simulink model "four_bots_CNN_DSM_7"  (R2018b)
settings: Solver=ode5  StartTime=0.0  StopTime=20.0  FixedStep=0.0002  RelTol=1e-3
(part 2 of 2)

== matlab function four_bots_CNN_DSM_7/Multi agent System NN & SMC/Agent 3/MATLAB Function ==
  data: agent_x1 input; x2_dot output; agent_x2 input; t input; control_input input; fx_dt output
function [x2_dot, fx_dt] = physical_model( agent_x1 , agent_x2, t, control_input )

Mass=[4,5,4,5];
Alpha=[0.087,0.090,0.085,0.092];
Radius=[0.18,0.20,0.24,0.22];
Inertia=[0.12,0.15,0.13,0.14];
Beta=[11.4,11.6,11.8,12.0];

%% assign the parameter according to serial number
serial_num = 3; 

m=Mass(serial_num);
alpha=Alpha(serial_num);
R=Radius(serial_num);
inertia=Inertia(serial_num);
beta=Beta(serial_num);

%% current states of the robot
dimension=3;

theta=agent_x1(dimension);

%% the real model of robot
M=diag([1/m,1/m,1/inertia]);
T=[-sin(theta), -sin(pi/3-theta), sin(pi/3+theta);
    cos(theta), -cos(pi/3-theta), -cos(pi/3+theta);
    R,          R,                  R];

real_fx = -beta*M*(T*T')*agent_x2;
uncertain = [0.3*sin(0.5*t)+2; 0.2*cos(0.5*t)+1.5; 0.1*sin(0.3*t)+1];

%% saturation is added here for convinience
Vmax=6; % the maximum voltage of the motor

u1up=Vmax/(alpha*m)*(abs(sin(theta))+abs(sin(pi/3-theta))+abs(sin(pi/3+theta)));
u1do=-Vmax/(alpha*m)*(abs(sin(theta))+abs(sin(pi/3-theta))+abs(sin(pi/3+theta)));
u2up=Vmax/(alpha*m)*(abs(cos(theta))+abs(cos(pi/3-theta))+abs(cos(pi/3+theta)));
u2do=-Vmax/(alpha*m)*(abs(cos(theta))+abs(cos(pi/3-theta))+abs(cos(pi/3+theta)));
u3up=R/(alpha*inertia)*3*Vmax;
u3do=-R/(alpha*inertia)*3*Vmax;

control_input(1) = max( min(control_input(1),u1up), u1do );
control_input(2) = max( min(control_input(2),u2up), u2do );
control_input(3) = max( min(control_input(3),u3up), u3do );


fx_dt=real_fx + uncertain; 

x2_dot = real_fx + control_input + uncertain;


end

== matlab function four_bots_CNN_DSM_7/Multi agent System NN & SMC/Agent 3/MATLAB Function1 ==
  data: fx_dt input; esti_error output; fx_dtdot input; E input
function esti_error = estimation_error(fx_dt, fx_dtdot, E)

c=2.5;
lambda=2.5;

esti_error = fx_dtdot + (c + lambda) * fx_dt - E; 

end

== matlab function four_bots_CNN_DSM_7/Multi agent System NN & SMC/Agent 4/Controller /Chebyshev Polynomials ==
  data: current_states input; phi_x output
function phi_x = Chebyshev_polynomials(current_states)

%% parameters that may alter
dimension=3;
cheby_order=3;

%% current states
x1=current_states(dimension*0+1:dimension*1);
x2=current_states(dimension*1+1:dimension*2);

%% initialization
phi_x=ones(1+2*dimension*cheby_order,1);

%% recursion procedure
now_x=[x1;x2];
for order = 1 : cheby_order
   if order == 1
      phi_x(2*dimension*(order-1)+2:2*dimension*order+1)=now_x;
   elseif order == 2
      phi_x(2*dimension*(order-1)+2:2*dimension*order+1)=2*now_x.*phi_x(2*dimension*(order-2)+2:2*dimension*(order-1)+1)-1;
   else
      phi_x(2*dimension*(order-1)+2:2*dimension*order+1)=2*now_x.*phi_x(2*dimension*(order-2)+2:2*dimension*(order-1)+1)-phi_x(2*dimension*(order-3)+2:2*dimension*(order-2)+1);
   end
end

end

== matlab function four_bots_CNN_DSM_7/Multi agent System NN & SMC/Agent 4/Controller /Control dot ==
  data: L input; E input; xi input; error input; u_dot output; reference input; u input
function u_dot = control_dot(L, E, xi, error, reference, u)

%% parameters that may change
dimension=3;
c=2.5;
lambda=2.5;
eta=80;

serial_num=4;

num_agent=size(L,1); 
%% codes
r_acc=reference(dimension*num_agent*2+1 : dimension*num_agent*3);
r_accdot=reference(dimension*num_agent*3+1 : dimension*num_agent*4);

xd2_dot = r_acc(dimension*(serial_num-1)+1 : dimension*serial_num);
xd2_ddot = r_accdot(dimension*(serial_num-1)+1 : dimension*serial_num);

e2=error(dimension*1+1:dimension*2);

u_dot= -E + xd2_ddot + (c+lambda)*xd2_dot - (c+lambda)*u -c*lambda*e2 - eta*xi;

end

== matlab function four_bots_CNN_DSM_7/Multi agent System NN & SMC/Agent 4/Controller /Error Calculation ==
  data: cur_states output; current_states input; L input; error output; reference input
function [cur_states , error] = error_calculation(current_states, L, reference)

%% parameters that may change for alternative use
dimension=3;
serial_num=4;

num_agent=size(L,1);
%% current states
% get current states
pos=current_states(dimension*num_agent*0+1 : dimension*num_agent*1);
vol=current_states(dimension*num_agent*1+1 : dimension*num_agent*2);
acc=current_states(dimension*num_agent*2+1 : dimension*num_agent*3);

% get current reference
r_pos=reference(dimension*num_agent*0+1 : dimension*num_agent*1);
r_vol=reference(dimension*num_agent*1+1 : dimension*num_agent*2);
r_acc=reference(dimension*num_agent*2+1 : dimension*num_agent*3);

% agent j's states
agent_x1 = pos(dimension*(serial_num-1)+1 : dimension*serial_num);
agent_x2 = vol(dimension*(serial_num-1)+1 : dimension*serial_num);

% agent_x2dot = acc(dimension*(serial_num-1)+1 : dimension*serial_num);
% 
% % agent j's reference
% r_x1=r_pos(dimension*(serial_num-1)+1 : dimension*serial_num);
% r_x2=r_vol(dimension*(serial_num-1)+1 : dimension*serial_num);
% r_x2dot=r_acc(dimension*(serial_num-1)+1 : dimension*serial_num);

e_1 = kron(L(serial_num, : ), eye(dimension) ) * (pos - r_pos);
e_2 = kron(L(serial_num, : ), eye(dimension) ) * (vol - r_vol);
e_2dot = kron(L(serial_num, : ), eye(dimension) ) * (acc - r_acc);

cur_states = [agent_x1;agent_x2];
error = [e_1 ; e_2 ; e_2dot];

end

== matlab function four_bots_CNN_DSM_7/Multi agent System NN & SMC/Agent 4/Controller /Estimation ==
  data: phi_x input; W input; E output
function E = estimation(phi_x, W)
%% estimation
E=W'*phi_x;

end

== matlab function four_bots_CNN_DSM_7/Multi agent System NN & SMC/Agent 4/Controller /Parameter Tuning ==
  data: phi_x input; xi input; W_dot output
function W_dot = parameter_tuning(phi_x, xi)

%% parameters that may alter
dimension=3;
cheby_order=3;
F=0.1*eye(1+2*dimension*cheby_order);

%% codes
W_dot = F*phi_x*xi';

end

== matlab function four_bots_CNN_DSM_7/Multi agent System NN & SMC/Agent 4/Controller /Sliding Variable Generation ==
  data: error input; xi output
function xi = sliding_variable(error)

%% parameters that may alter
dimension=3;
c=2.5;
lambda=2.5;

%% codes
error_1=error(dimension*0+1:dimension*1);
error_2=error(dimension*1+1:dimension*2);
error_2dot=error(dimension*2+1:dimension*3);

xi = error_2dot + (c + lambda)* error_2 + lambda * c * error_1;

end

== matlab function four_bots_CNN_DSM_7/Multi agent System NN & SMC/Agent 4/Controller /neural_initial ==
  data: weight output
function weight = neural_initialize()

% cheby_order   : order of chebyshev polynomials
% dimension     : dimension of the system

cheby_order=3;
dimension=3;

weight = zeros(1+2*cheby_order*dimension, dimension);

end

== matlab function four_bots_CNN_DSM_7/Multi agent System NN & SMC/Agent 4/MATLAB Function ==
  data: agent_x1 input; x2_dot output; agent_x2 input; t input; control_input input; fx_dt output
function [x2_dot, fx_dt] = physical_model( agent_x1 , agent_x2, t, control_input )

Mass=[4,5,4,5];
Alpha=[0.087,0.090,0.085,0.092];
Radius=[0.18,0.20,0.24,0.22];
Inertia=[0.12,0.15,0.13,0.14];
Beta=[11.4,11.6,11.8,12.0];

%% assign the parameter according to serial number
serial_num = 4; 

m=Mass(serial_num);
alpha=Alpha(serial_num);
R=Radius(serial_num);
inertia=Inertia(serial_num);
beta=Beta(serial_num);

%% current states of the robot
dimension=3;

theta=agent_x1(dimension);

%% the real model of robot
M=diag([1/m,1/m,1/inertia]);
T=[-sin(theta), -sin(pi/3-theta), sin(pi/3+theta);
    cos(theta), -cos(pi/3-theta), -cos(pi/3+theta);
    R,          R,                  R];

real_fx = -beta*M*(T*T')*agent_x2;
uncertain = [0.3*sin(0.5*t)+2; 0.2*cos(0.5*t)+1.5; 0.1*sin(0.3*t)+1];

%% saturation is added here for convinience
Vmax=6; % the maximum voltage of the motor

u1up=Vmax/(alpha*m)*(abs(sin(theta))+abs(sin(pi/3-theta))+abs(sin(pi/3+theta)));
u1do=-Vmax/(alpha*m)*(abs(sin(theta))+abs(sin(pi/3-theta))+abs(sin(pi/3+theta)));
u2up=Vmax/(alpha*m)*(abs(cos(theta))+abs(cos(pi/3-theta))+abs(cos(pi/3+theta)));
u2do=-Vmax/(alpha*m)*(abs(cos(theta))+abs(cos(pi/3-theta))+abs(cos(pi/3+theta)));
u3up=R/(alpha*inertia)*3*Vmax;
u3do=-R/(alpha*inertia)*3*Vmax;

control_input(1) = max( min(control_input(1),u1up), u1do );
control_input(2) = max( min(control_input(2),u2up), u2do );
control_input(3) = max( min(control_input(3),u3up), u3do );


fx_dt=real_fx + uncertain; 

x2_dot = real_fx + control_input + uncertain;


end

== matlab function four_bots_CNN_DSM_7/Multi agent System NN & SMC/Agent 4/MATLAB Function1 ==
  data: fx_dt input; esti_error output; fx_dtdot input; E input
function esti_error = estimation_error(fx_dt, fx_dtdot, E)

c=2.5;
lambda=2.5;

esti_error = fx_dtdot + (c + lambda) * fx_dt - E; 

end

== matlab function four_bots_CNN_DSM_7/Reference Generator1/Acceleration reference ==
  data: t input; x2d_dot output
function x2d_dot = gene_ref_x2_dot(t)

%% generate position reference
radius=3;
w=0.1;
phase=-pi/4;

x1=[-radius*w^2*cos(w*t+pi/2*0+phase); -radius*w^2*sin(w*t+pi/2*0+phase); 0];
x2=[-radius*w^2*cos(w*t+pi/2*1+phase); -radius*w^2*sin(w*t+pi/2*1+phase); 0];
x3=[-radius*w^2*cos(w*t+pi/2*2+phase); -radius*w^2*sin(w*t+pi/2*2+phase); 0];
x4=[-radius*w^2*cos(w*t+pi/2*3+phase); -radius*w^2*sin(w*t+pi/2*3+phase); 0];

x2d_dot=[x1;x2;x3;x4];

== matlab function four_bots_CNN_DSM_7/Reference Generator1/Acceleration_dot Reference ==
  data: t input; x2ddot output
function x2ddot = gene_ref_x2ddot(t)

%% generate position reference
radius=3;
w=0.1;
phase=-pi/4;

x1=[radius*w^3*sin(w*t+pi/2*0+phase); -radius*w^3*cos(w*t+pi/2*0+phase); 0];
x2=[radius*w^3*sin(w*t+pi/2*1+phase); -radius*w^3*cos(w*t+pi/2*1+phase); 0];
x3=[radius*w^3*sin(w*t+pi/2*2+phase); -radius*w^3*cos(w*t+pi/2*2+phase); 0];
x4=[radius*w^3*sin(w*t+pi/2*3+phase); -radius*w^3*cos(w*t+pi/2*3+phase); 0];

x2ddot=[x1;x2;x3;x4];

== matlab function four_bots_CNN_DSM_7/Reference Generator1/Position Reference ==
  data: t input; x1d output
function x1d = gene_ref_x1(t)

%% generate position reference
radius=3;
w=0.1;
bias_x=0;
bias_y=0;
phase=-pi/4;

x1=[radius*cos(w*t+pi/2*0+phase)+bias_x ; radius*sin(w*t+pi/2*0+phase)+bias_y ; 0];
x2=[radius*cos(w*t+pi/2*1+phase)+bias_x ; radius*sin(w*t+pi/2*1+phase)+bias_y ; 0];
x3=[radius*cos(w*t+pi/2*2+phase)+bias_x ; radius*sin(w*t+pi/2*2+phase)+bias_y ; 0];
x4=[radius*cos(w*t+pi/2*3+phase)+bias_x ; radius*sin(w*t+pi/2*3+phase)+bias_y ; 0];

x1d=[x1;x2;x3;x4];

== matlab function four_bots_CNN_DSM_7/Reference Generator1/Speed Reference ==
  data: t input; x2d output
function x2d = gene_ref_x2(t)

%% generate position reference
radius=3;
w=0.1;
phase=-pi/4;

x1=[-radius*w*sin(w*t+pi/2*0+phase); radius*w*cos(w*t+pi/2*0+phase); 0];
x2=[-radius*w*sin(w*t+pi/2*1+phase); radius*w*cos(w*t+pi/2*1+phase); 0];
x3=[-radius*w*sin(w*t+pi/2*2+phase); radius*w*cos(w*t+pi/2*2+phase); 0];
x4=[-radius*w*sin(w*t+pi/2*3+phase); radius*w*cos(w*t+pi/2*3+phase); 0];

x2d=[x1;x2;x3;x4];

== matlab function four_bots_CNN_DSM_7/Multi agent System NN & SMC/Agent 3/Controller /Hysteresis/MATLAB Function1 ==
  data: u input; output output; u_dot input; zeta input; zeta_dot output
function [output,zeta_dot] = B_W_hysteresis(u, u_dot, zeta)

mu_1=1.5;
mu_2=3;
beta=1;
chi=0.5;
n=2;

output=mu_1*u+mu_2*zeta;

f=ones(3,1)-beta*sign(u_dot).*abs(zeta).^(n-1).*zeta-chi*abs(zeta).^n;

zeta_dot=u_dot.*f;
end

== matlab function four_bots_CNN_DSM_7/Multi agent System NN & SMC/Agent 3/Controller /Hysteresis/MATLAB Function2 ==
  data: u input; output output; u_dot input; zeta_1 input; zeta1_dot output
function [output,zeta1_dot] = inv_B_W_hysteresis(u, u_dot, zeta_1)

mu_1=1.5;
mu_2=3;
beta=1;
chi=0.5;
n=2;

output=1/mu_1*u - mu_2/mu_1*zeta_1;

f=ones(3,1)-beta*sign(u_dot/mu_1).*abs(zeta_1).^(n-1).*zeta_1-chi*abs(zeta_1).^n;

zeta1_dot=u_dot.*f./(mu_1+mu_2*f);
end

== matlab function four_bots_CNN_DSM_7/Multi agent System NN & SMC/Agent 1 /Controller /MATLAB Function ==
  data: W input; W output
function W = smooth_projection(W)

%% smooth projection
Wmax=0.3;
Wmin=-0.3;
epsi=0.01;

for i=1:size(W,1)
   for j=1:size(W,2)
      if W(i,j)>Wmax
          W(i,j)=Wmax + epsi * (1-exp(-(W(i,j)-Wmax)/epsi));
      elseif W(i,j)<Wmin
          W(i,j)=Wmin - epsi * (1-exp((W(i,j)-Wmin)/epsi));
      else
          W(i,j)=W(i,j);
      end
   end
end

end

== matlab function four_bots_CNN_DSM_7/Multi agent System NN & SMC/Agent 2/Controller /MATLAB Function ==
  data: W input; W output
function W = smooth_projection(W)

%% smooth projection
Wmax=0.3;
Wmin=-0.3;
epsi=0.01;

for i=1:size(W,1)
   for j=1:size(W,2)
      if W(i,j)>Wmax
          W(i,j)=Wmax + epsi * (1-exp(-(W(i,j)-Wmax)/epsi));
      elseif W(i,j)<Wmin
          W(i,j)=Wmin - epsi * (1-exp((W(i,j)-Wmin)/epsi));
      else
          W(i,j)=W(i,j);
      end
   end
end

end

== matlab function four_bots_CNN_DSM_7/Multi agent System NN & SMC/Agent 4/Controller /Hysteresis1/MATLAB Function1 ==
  data: u input; output output; u_dot input; zeta input; zeta_dot output
function [output,zeta_dot] = B_W_hysteresis(u, u_dot, zeta)

mu_1=1.5;
mu_2=3;
beta=1;
chi=0.5;
n=2;

output=mu_1*u+mu_2*zeta;

f=ones(3,1)-beta*sign(u_dot).*abs(zeta).^(n-1).*zeta-chi*abs(zeta).^n;

zeta_dot=u_dot.*f;
end

== matlab function four_bots_CNN_DSM_7/Multi agent System NN & SMC/Agent 4/Controller /Hysteresis1/MATLAB Function2 ==
  data: u input; output output; u_dot input; zeta_1 input; zeta1_dot output
function [output,zeta1_dot] = inv_B_W_hysteresis(u, u_dot, zeta_1)

mu_1=1.5;
mu_2=3;
beta=1;
chi=0.5;
n=2;

output=1/mu_1*u - mu_2/mu_1*zeta_1;

f=ones(3,1)-beta*sign(u_dot/mu_1).*abs(zeta_1).^(n-1).*zeta_1-chi*abs(zeta_1).^n;

zeta1_dot=u_dot.*f./(mu_1+mu_2*f);
end

== matlab function four_bots_CNN_DSM_7/Multi agent System NN & SMC/Agent 3/Controller /MATLAB Function ==
  data: W input; W output
function W = smooth_projection(W)

%% smooth projection
Wmax=0.3;
Wmin=-0.3;
epsi=0.01;

for i=1:size(W,1)
   for j=1:size(W,2)
      if W(i,j)>Wmax
          W(i,j)=Wmax + epsi * (1-exp(-(W(i,j)-Wmax)/epsi));
      elseif W(i,j)<Wmin
          W(i,j)=Wmin - epsi * (1-exp((W(i,j)-Wmin)/epsi));
      else
          W(i,j)=W(i,j);
      end
   end
end

end

== matlab function four_bots_CNN_DSM_7/Multi agent System NN & SMC/Agent 4/Controller /MATLAB Function ==
  data: W input; W output
function W = smooth_projection(W)

%% smooth projection
Wmax=0.3;
Wmin=-0.3;
epsi=0.01;

for i=1:size(W,1)
   for j=1:size(W,2)
      if W(i,j)>Wmax
          W(i,j)=Wmax + epsi * (1-exp(-(W(i,j)-Wmax)/epsi));
      elseif W(i,j)<Wmin
          W(i,j)=Wmin - epsi * (1-exp((W(i,j)-Wmin)/epsi));
      else
          W(i,j)=W(i,j);
      end
   end
end

end
